simulink model "ThreeFeeder"  (R2023b)
settings: Solver=FixedStepDiscrete  StartTime=0.0  StopTime=2  RelTol=1e-3
InitFcn:
  | Frequency = 50;
  | w = 2*pi*Frequency;
  | 
  | Vnom_ph_ph = 22000;
  | Vnom = Vnom_ph_ph/sqrt(3);
  | 
  | % miles/km
  | mi2km = 1.60934;
  | % feet to km
  | ft2km = 0.0003048;
  | % microsiemens to Farads
  | ms2F = 1/2/pi/60*1e-6;
  | 
  | % Breaker
  | NOP1 = 0;
  | NOP2 = 0;
  | NOP3 = 0;
  | Fault = 0;
  | CB1 = 1;
  | CB2 = 1;
  | CB3 = 1;
undefined symbols (not defined in the file): Angle, D11, Delta, Magnitude
libraries: spsLoadFlowBusLib x24, spsThreePhasePISectionLineLib x22, spsThreePhaseVIMeasurementLib x21, spsThreePhaseSeriesRLCLoadLib x18, spsCurrentMeasurementLib x9, spsGroundLib x9, spsVoltageMeasurementLib x9, spsThreePhaseBreakerLib x6, spsThreePhaseSeriesRLCBranchLib x6, spsThreePhaseSourceLib x4, spsThreePhaseTransformerTwoWindingsLib x3, spsThreePhaseFaultLib x1
(part 2 of 2)

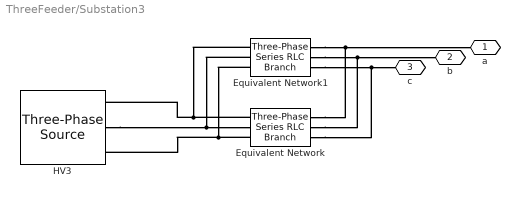
== system ThreeFeeder/Substation3 ==
  Equivalent Network : spsThreePhaseSeriesRLCBranchLib/Three-Phase Series RLC Branch  LConnTagsString=A|B|C  RConnTagsString=A|B|C  BranchType=RL  Resistance=5  Inductance=1  Capacitance=1.0  Measurements=None
  Equivalent Network1 : spsThreePhaseSeriesRLCBranchLib/Three-Phase Series RLC Branch  LConnTagsString=A|B|C  RConnTagsString=A|B|C  BranchType=C  Resistance=5  Inductance=1  Capacitance=1  Measurements=None
  HV3 : spsThreePhaseSourceLib/Three-Phase Source  InternalConnection=Yg  VoltagePhases=off  Voltage=120e3  PhaseAngle=0  Voltage_phases=[1 1 1]*(115e3)/sqrt(3)  PhaseAngles_phases=[0 -120 +120]  Frequency=Frequency  NonIdealSource=off  SpecifyImpedance=on  Resistance=0.8929  Inductance=16.58e-3  ShortCircuitLevel=Apparent_power_gen1  BaseVoltage=Vnom_ph_ph  XRratio=8  BusType=PV  Pref=1000e6  Qref=0  Prefabc=[10e3, 10e3, 10e3]  Qrefabc=[0, 0, 0]  Qmin=[-1500 -1500 -1500]*1e6  Qmax=[1500 1500 1500]*1e6
  a : PMIOPort  Side=Right
  b : PMIOPort  Port=2  Side=Right
  c : PMIOPort  Port=3  Side=Right
  connections:
  Equivalent Network/LConn3 -- Equivalent Network1/LConn3 -- HV3/RConn3
  HV3/RConn2 -- Equivalent Network1/LConn2 -- Equivalent Network/LConn2
  Equivalent Network/LConn1 -- Equivalent Network1/LConn1 -- HV3/RConn1
  Equivalent Network1/RConn2 -- Equivalent Network/RConn2 -- b/RConn1
  Equivalent Network1/RConn1 -- Equivalent Network/RConn1 -- a/RConn1
  Equivalent Network1/RConn3 -- Equivalent Network/RConn3 -- c/RConn1
